simulink model "Sim_Exemplo_5_4_1"  (R2013b)
settings: Solver=ode45  StartTime=0.0  StopTime=10.0  RelTol=1e-3
values from neighbouring files (symbols this model uses):
  A = [ -1.01887    0.90506 ... (first row only)    [Example_5_4_1_Lewis.m]
  B = [ -0.00215 ... (first row only)    [Example_5_4_1_Lewis.m]
  C = [  57.2988          0 ... (first row only)    [Example_5_4_1_Lewis.m]    (also in Main.m = x(1)*tf([1 x(2)],[1 1]); fnCost.m = x(1)*tf([1 x(2)],[1 1]))
  D = [        0 ... (first row only)    [Example_5_4_1_Lewis.m]
  x = fminsearch(Custo, x0, options)    [Example_5_4_1_Lewis.m]    (also in Main.m = fminsearch(@fnCost, x0, options))
settings Model: Creator=Eduardo  LastModifiedBy=Eduardo

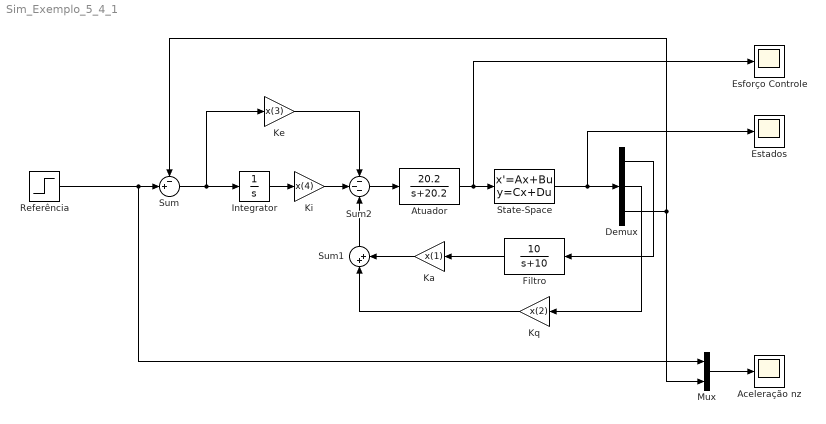
== system Sim_Exemplo_5_4_1 ==
  Aceleração nz : Scope
      settings: SaveName=ScopeData2
  Atuador : TransferFcn  Numerator=[20.2]  Denominator=[1 20.2]
  Demux : Demux  Outputs=3
  Esforço Controle : Scope
  Estados : Scope
  Filtro : TransferFcn  Numerator=[10]  Denominator=[1 10]
  Integrator : Integrator
  Ka : Gain  Gain=x(1)
  Ke : Gain  Gain=x(3)
  Ki : Gain  Gain=x(4)
  Kq : Gain  Gain=x(2)
  Mux : Mux  Inputs=2
  Referência : Step  SampleTime=0
  State-Space : StateSpace  A=A  B=B  C=C  D=D  X0=0
  Sum : Sum  Inputs=-+|
  Sum1 : Sum  Inputs=|++
  Sum2 : Sum  Inputs=---
  wires:
  Atuador/1 -> Esforço Controle/1, State-Space/1
  State-Space/1 -> Estados/1, Demux/1
  Demux/2 -> Kq/1
  Demux/1 -> Filtro/1
  Integrator/1 -> Ki/1
  Sum/1 -> Ke/1, Integrator/1
  Demux/3 -> Mux/2, Sum/1
  Filtro/1 -> Ka/1
  Kq/1 -> Sum1/1
  Ka/1 -> Sum1/2
  Sum2/1 -> Atuador/1
  Ke/1 -> Sum2/1
  Ki/1 -> Sum2/2
  Sum1/1 -> Sum2/3
  Mux/1 -> Aceleração nz/1
  Referência/1 -> Mux/1, Sum/2
